simulink model "CAES_storage"  (R2026a)
settings: Solver=VariableStepAuto  StopTime=500
settings Model: Creator=milenadaniltsenko  LastModifiedBy=milenadaniltsenko

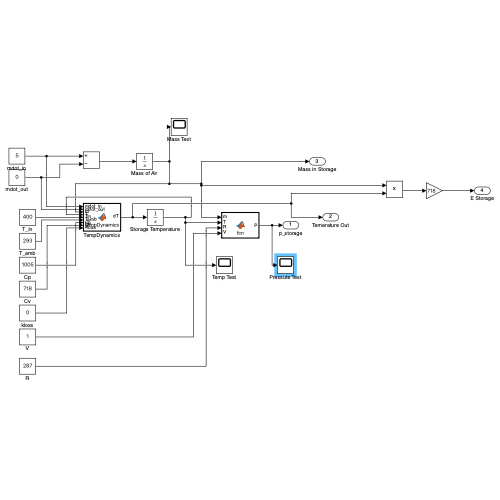
[thumbnail: Simulink's stored preview of the top-level diagram]
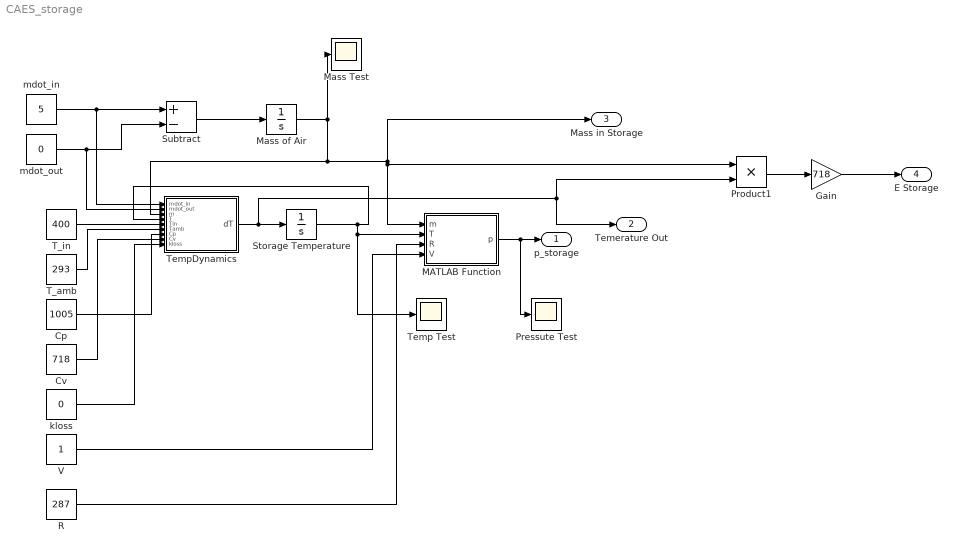
== system CAES_storage ==
  Cp : Constant  Value=1005
  Cv : Constant  Value=718
  Gain : Gain  Gain=718
  MATLAB Function : MATLAB Function  TreatAsAtomicUnit=on
  Mass Test : Scope
      settings: ActiveDisplayYMinimum=-1  ActiveDisplayYMaximum=1
  Mass of Air : Integrator  InitialCondition=10
  Pressute Test : Scope
      settings: ActiveDisplayYMinimum=-3.2534701809240017E+9  ActiveDisplayYMaximum=1.0291728329865596E+9
  Product1 : Product
  R : Constant  Value=287
  Storage Temperature : Integrator  InitialCondition=293
  Subtract : Sum  Inputs=+-
  T_amb : Constant  Value=293
  T_in : Constant  Value=400
  Temp Test : Scope
      settings: ActiveDisplayYMinimum=-1  ActiveDisplayYMaximum=1  DataLoggingVariableName=ScopeData2
  TempDynamics : MATLAB Function  TreatAsAtomicUnit=on
  V : Constant
  kloss : Constant  Value=0
  mdot_in : Constant  Value=5
  mdot_out : Constant  Value=0
  p_storage : Outport
  Temerature Out : Outport  Port=2
  Mass in Storage : Outport  Port=3
  E Storage : Outport  Port=4
  wires:
  mdot_out/1 -> TempDynamics/2(mdot_out), Subtract/2
  Subtract/1 -> Mass of Air/1
  T_in/1 -> TempDynamics/5(Tin)
  T_amb/1 -> TempDynamics/6(Tamb)
  Cp/1 -> TempDynamics/7(Cp)
  Cv/1 -> TempDynamics/8(Cv)
  kloss/1 -> TempDynamics/9(kloss)
  V/1 -> MATLAB Function/4(V)
  TempDynamics/1(dT) -> Temerature Out/1, Product1/2, Storage Temperature/1
  R/1 -> MATLAB Function/3(R)
  MATLAB Function/1(p) -> Pressute Test/1, p_storage/1
  Product1/1 -> Gain/1
  mdot_in/1 -> TempDynamics/1(mdot_in), Subtract/1
  Gain/1 -> E Storage/1
  Mass of Air/1 -> Mass Test/1, Product1/1, MATLAB Function/1(m), Mass in Storage/1, TempDynamics/3(m)
  Storage Temperature/1 -> MATLAB Function/2(T), Temp Test/1, TempDynamics/4(T)

== matlab function CAES_storage/TempDynamics ==
  data: mdot_in input; dT output; mdot_out input; m input; T input; Tin input; Tamb input; Cp input; Cv input; kloss input
function dT = tempDynamics(mdot_in, mdot_out, m, T, Tin, Tamb, Cp, Cv, kloss)
% m: mass of air in tank
% T: current temperature of air in tank
% Tin: temperature of air coming in
% Cv: Specific heat at constant volume (~718 J/kgK)
% Cp: Specific heat at constant pressure (~1005 J/kgK)

if m <= 0.01 % Use a small threshold to avoid division by zero
    dT = 0;
else
    % Energy balance: d(m*Cv*T)/dt = m_in*h_in - m_out*h_out - Q_loss
    % Solving for dT/dt results in
    
    dm_dt = mdot_in - mdot_out;
    dT = ( (mdot_in * Cp * Tin) - (mdot_out * Cp * T) - (dm_dt * Cv * T) - (kloss * (T - Tamb)) ) / (m * Cv);
end

== matlab function CAES_storage/MATLAB Function ==
  data: m input; p output; T input; R input; V input
function p = fcn(m, T, R, V)
    p = (m * R * T) / V;
end
